simulink model "sampleModel1882"  (R2023a)
settings: Solver=VariableStepAuto  StartTime=0.0  StopTime=10.0  RelTol=1e-3
libraries: hdlsllib x4, simulink x1
settings Model: Creator=user1  LastModifiedBy=user1

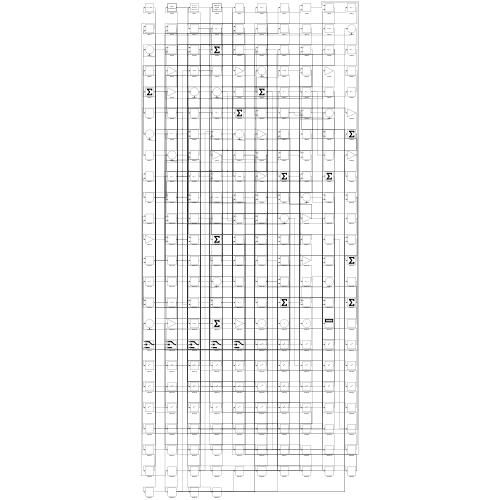
[thumbnail: Simulink's stored preview of the top-level diagram]
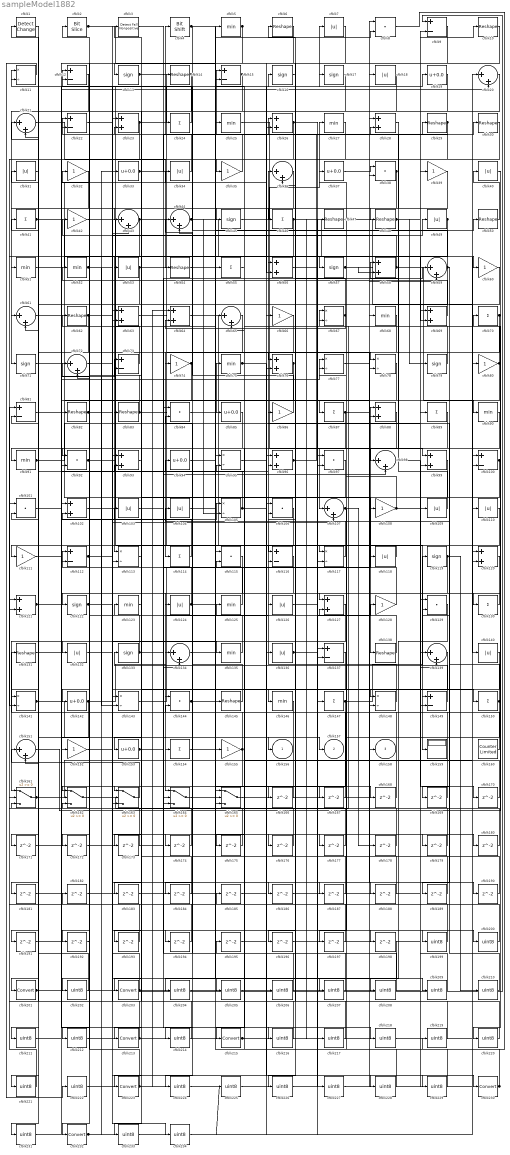
== system sampleModel1882 ==
  cfblk1 : simulink/Logic and Bit Operations/Detect Change  vinit=0  OutDataTypeStr=boolean
      settings: LibrarySourceBlock=|
      | hdlsllib/Logic and Bit
      | Operations/Detect
      | Change
  cfblk{6,10,14,29..30,47..48,50,54,62,82..83,131,138,145} (15 alike) : Reshape
  cfblk{9,12,15,22,73,81,100,112,116,137,149} (11 alike) : Sum  Inputs=+-
  cfblk{8,38,84,92,97,101,106,115,129,144} (10 alike) : DotProduct  OutDataTypeStr=Inherit: Inherit via internal rule
  cfblk{23,26,28,56,58,63..64,69,76,88,93,96,99,102,120..121,127} (17 alike) : Sum
  cfblk{7,18,31,34,40,49,53,103..104,109..110,118,124,126,132,136,140} (17 alike) : Abs  SaturateOnIntegerOverflow=off
  cfblk{11,67,77..78,95,105,113,117,141,143,148} (11 alike) : Product  Inputs=*/  RndMeth=Zero  SaturateOnIntegerOverflow=on
  cfblk{20..21,36,43..44,59,61,65,72,98,107,134,139,151} (14 alike) : Sum  Inputs=|++
  cfblk{32,35,39,42,60,66,74,80,86,108,111,128,152,155} (14 alike) : Gain
  cfblk{24,41,46,55,70,87,89,114,130,147,150,154} (12 alike) : Sum  Inputs=+
  cfblk{13,16..17,45,57,71,79,119,122,133} (10 alike) : Signum
  cfblk{5,25,27,51..52,68,75,90..91,123,125,135,146} (13 alike) : MinMax
  cfblk{19,33,37,85,94,142,153} (7 alike) : Bias  Bias=0.0  SaturateOnIntegerOverflow=off
  cfblk159 : Display
  cfblk160 : hdlsllib/Sources/Counter Limited  uplimit=7  tsamp=-1
  cfblk{161..165} (5 alike) : Switch  SaturateOnIntegerOverflow=off  InputSameDT=off
  cfblk{166..198} (33 alike) : Delay  SampleTime=1
  cfblk{199..200,202,204..212,214,216..222,224..229,231,233..234} (29 alike) : DataTypeConversion  OutDataTypeStr=uint8  SaturateOnIntegerOverflow=off  RndMeth=Floor
  cfblk2 : hdlsllib/Logic and Bit Operations/Bit Slice  lidx=7  ridx=0
  cfblk{201,203,213,215,223,230,232} (7 alike) : DataTypeConversion  SaturateOnIntegerOverflow=off  RndMeth=Floor
  cfblk3 : hdlsllib/Logic and Bit Operations/Detect Fall Nonpositive  vinit=0  OutDataTypeStr=boolean
  cfblk4 : hdlsllib/Logic and Bit Operations/Bit Shift  mode=Shift Left Logical  N=0
  cfblk156 : Outport  VectorParamsAs1DForOutWhenUnconnected=off
  cfblk157 : Outport  Port=2  VectorParamsAs1DForOutWhenUnconnected=off
  cfblk158 : Outport  Port=3  VectorParamsAs1DForOutWhenUnconnected=off
  wires:
  cfblk127/1 -> cfblk161/1
  cfblk58/1 -> cfblk90/1, cfblk42/1
  cfblk42/1 -> cfblk117/1
  cfblk107/1 -> cfblk133/1, cfblk178/1
  cfblk12/1 -> cfblk71/1
  cfblk162/1 -> cfblk67/1
  cfblk96/1 -> cfblk30/1, cfblk196/1
  cfblk10/1 -> cfblk13/1
  cfblk50/1 -> cfblk40/1
  cfblk5/1 -> cfblk122/1, cfblk112/2
  cfblk150/1 -> cfblk86/1, cfblk104/1, cfblk197/1
  cfblk91/1 -> cfblk88/1, cfblk9/2, cfblk96/2
  cfblk25/1 -> cfblk99/1
  cfblk64/1 -> cfblk159/1
  cfblk151/1 -> cfblk70/1
  cfblk49/1 -> cfblk113/1, cfblk69/2
  cfblk71/1 -> cfblk138/1
  cfblk92/1 -> cfblk7/1, cfblk14/1
  cfblk17/1 -> cfblk132/1
  cfblk66/1 -> cfblk114/1
  cfblk148/1 -> cfblk36/1
  cfblk124/1 -> cfblk5/1, cfblk73/2
  cfblk40/1 -> cfblk130/1
  cfblk84/1 -> cfblk75/1
  cfblk80/1 -> cfblk22/1, cfblk148/2
  cfblk145/1 -> cfblk102/2
  cfblk141/1 -> cfblk157/1, cfblk77/2
  cfblk134/1 -> cfblk65/1
  cfblk120/1 -> cfblk232/1
  cfblk163/1 -> cfblk151/1
  cfblk106/1 -> cfblk215/1
  cfblk44/1 -> cfblk57/1, cfblk105/2
  cfblk117/1 -> cfblk56/1
  cfblk114/1 -> cfblk32/1
  cfblk119/1 -> cfblk164/1, cfblk210/1
  cfblk142/1 -> cfblk126/1, cfblk191/1
  cfblk54/1 -> cfblk55/1
  cfblk94/1 -> cfblk155/1
  cfblk147/1 -> cfblk119/1, cfblk192/1
  cfblk7/1 -> cfblk146/1
  cfblk83/1 -> cfblk165/1, cfblk62/1
  cfblk102/1 -> cfblk50/1
  cfblk34/1 -> cfblk4/1
  cfblk47/1 -> cfblk100/1
  cfblk133/1 -> cfblk112/1, cfblk177/1
  cfblk43/1 -> cfblk78/1, cfblk141/2
  cfblk165/1 -> cfblk8/1
  cfblk45/1 -> cfblk27/1
  cfblk23/1 -> cfblk16/1, cfblk121/2
  cfblk13/1 -> cfblk76/1, cfblk216/1
  cfblk152/1 -> cfblk230/1
  cfblk41/1 -> cfblk117/2, cfblk97/2
  cfblk19/1 -> cfblk63/2
  cfblk115/1 -> cfblk203/1
  cfblk121/1 -> cfblk154/1, cfblk34/1, cfblk105/1
  cfblk137/1 -> cfblk223/1
  cfblk139/1 -> cfblk148/1
  cfblk95/1 -> cfblk136/1
  cfblk128/1 -> cfblk2/1
  cfblk109/1 -> cfblk24/1
  cfblk122/1 -> cfblk186/1, cfblk187/1
  cfblk153/1 -> cfblk59/1, cfblk118/1
  cfblk143/1 -> cfblk88/2
  cfblk70/1 -> cfblk116/1, cfblk72/2
  cfblk1/1 -> cfblk201/1
  cfblk85/1 -> cfblk113/2
  cfblk2/1 -> cfblk85/1, cfblk194/1
  cfblk100/1 -> cfblk165/2, cfblk220/1
  cfblk62/1 -> cfblk135/1, cfblk181/1
  cfblk53/1 -> cfblk165/3, cfblk98/2, cfblk171/1
  cfblk112/1 -> cfblk49/1, cfblk172/1, cfblk176/1
  cfblk48/1 -> cfblk98/1, cfblk79/1, cfblk10/1
  cfblk38/1 -> cfblk44/2, cfblk183/1
  cfblk93/1 -> cfblk23/2
  cfblk67/1 -> cfblk26/1, cfblk64/2
  cfblk46/1 -> cfblk100/2, cfblk141/1, cfblk217/1
  cfblk21/1 -> cfblk54/1
  cfblk118/1 -> cfblk111/1
  cfblk22/1 -> cfblk108/1
  cfblk37/1 -> cfblk38/1
  cfblk35/1 -> cfblk15/1
  cfblk36/1 -> cfblk45/1
  cfblk155/1 -> cfblk131/1, cfblk184/1
  cfblk87/1 -> cfblk124/1, cfblk59/2
  cfblk154/1 -> cfblk8/2
  cfblk61/1 -> cfblk158/1
  cfblk63/1 -> cfblk145/1
  cfblk144/1 -> cfblk156/1, cfblk209/1
  cfblk130/1 -> cfblk127/1
  cfblk33/1 -> cfblk60/1, cfblk29/1
  cfblk75/1 -> cfblk87/1, cfblk207/1
  cfblk105/1 -> cfblk41/1, cfblk200/1
  cfblk29/1 -> cfblk61/1, cfblk53/1, cfblk28/2
  cfblk51/1 -> cfblk17/1
  cfblk78/1 -> cfblk164/2
  cfblk76/1 -> cfblk83/1, cfblk92/2
  cfblk28/1 -> cfblk48/1
  cfblk69/1 -> cfblk52/1
  cfblk57/1 -> cfblk140/1, cfblk58/2
  cfblk26/1 -> cfblk78/2, cfblk35/1
  cfblk79/1 -> cfblk58/1
  cfblk73/1 -> cfblk12/1
  cfblk52/1 -> cfblk143/2, cfblk174/1
  cfblk24/1 -> cfblk11/1
  cfblk90/1 -> cfblk107/1
  cfblk14/1 -> cfblk43/1, cfblk142/1
  cfblk140/1 -> cfblk164/3
  cfblk101/1 -> cfblk19/1
  cfblk32/1 -> cfblk51/1
  cfblk4/1 -> cfblk134/1, cfblk150/1
  cfblk131/1 -> cfblk20/2
  cfblk160/1 -> cfblk11/2
  cfblk161/1 -> cfblk80/1, cfblk31/1
  cfblk86/1 -> cfblk44/1
  cfblk9/1 -> cfblk46/1
  cfblk27/1 -> cfblk163/3
  cfblk138/1 -> cfblk125/1
  cfblk59/1 -> cfblk61/2, cfblk12/2, cfblk189/1
  cfblk15/1 -> cfblk21/2, cfblk92/1
  cfblk132/1 -> cfblk43/2
  cfblk123/1 -> cfblk213/1
  cfblk135/1 -> cfblk103/1
  cfblk149/1 -> cfblk6/1
  cfblk97/1 -> cfblk144/1
  cfblk108/1 -> cfblk139/1, cfblk67/2, cfblk77/1
  cfblk31/1 -> cfblk91/1
  cfblk55/1 -> cfblk25/1
  cfblk125/1 -> cfblk72/1
  cfblk65/1 -> cfblk74/1
  cfblk111/1 -> cfblk73/1
  cfblk82/1 -> cfblk149/1, cfblk107/2, cfblk205/1
  cfblk74/1 -> cfblk162/1, cfblk153/1
  cfblk136/1 -> cfblk128/1, cfblk229/1
  cfblk6/1 -> cfblk56/2
  cfblk16/1 -> cfblk166/1
  cfblk166/1 -> cfblk163/1
  cfblk110/1 -> cfblk167/1
  cfblk167/1 -> cfblk101/2
  cfblk164/1 -> cfblk168/1
  cfblk168/1 -> cfblk102/1
  cfblk60/1 -> cfblk169/1
  cfblk169/1 -> cfblk116/2
  cfblk98/1 -> cfblk170/1
  cfblk170/1 -> cfblk15/2
  cfblk171/1 -> cfblk134/2
  cfblk113/1 -> cfblk173/1
  cfblk173/1 -> cfblk22/2
  cfblk174/1 -> cfblk163/2
  cfblk88/1 -> cfblk175/1
  cfblk175/1 -> cfblk151/2
  cfblk176/1 -> cfblk65/2
  cfblk177/1 -> cfblk161/2
  cfblk178/1 -> cfblk127/2
  cfblk56/1 -> cfblk179/1
  cfblk179/1 -> cfblk63/1
  cfblk103/1 -> cfblk180/1
  cfblk180/1 -> cfblk21/1
  cfblk181/1 -> cfblk26/2
  cfblk183/1 -> cfblk76/2
  cfblk184/1 -> cfblk93/2
  cfblk186/1 -> cfblk99/2
  cfblk187/1 -> cfblk144/2
  cfblk72/1 -> cfblk188/1
  cfblk188/1 -> cfblk36/2
  cfblk189/1 -> cfblk97/1
  cfblk77/1 -> cfblk190/1
  cfblk190/1 -> cfblk28/1
  cfblk191/1 -> cfblk162/2
  cfblk192/1 -> cfblk162/3
  cfblk18/1 -> cfblk193/1
  cfblk193/1 -> cfblk23/1
  cfblk194/1 -> cfblk161/3
  cfblk196/1 -> cfblk139/2
  cfblk197/1 -> cfblk121/1
  cfblk104/1 -> cfblk198/1
  cfblk3/1 -> cfblk199/1
  cfblk199/1 -> cfblk94/1
  cfblk200/1 -> cfblk3/1
  cfblk201/1 -> cfblk69/1, cfblk109/1
  cfblk182/1 -> cfblk202/1
  cfblk202/1 -> cfblk1/1
  cfblk203/1 -> cfblk9/1, cfblk93/1
  cfblk198/1 -> cfblk204/1
  cfblk204/1 -> cfblk115/1
  cfblk205/1 -> cfblk115/2
  cfblk185/1 -> cfblk206/1
  cfblk206/1 -> cfblk84/1
  cfblk207/1 -> cfblk185/1
  cfblk129/1 -> cfblk208/1
  cfblk208/1 -> cfblk84/2
  cfblk209/1 -> cfblk129/1
  cfblk210/1 -> cfblk129/2
  cfblk89/1 -> cfblk211/1
  cfblk211/1 -> cfblk82/1
  cfblk116/1 -> cfblk212/1
  cfblk212/1 -> cfblk89/1
  cfblk213/1 -> cfblk149/2, cfblk143/1
  cfblk20/1 -> cfblk214/1
  cfblk214/1 -> cfblk123/1
  cfblk215/1 -> cfblk18/1, cfblk147/1
  cfblk216/1 -> cfblk106/1
  cfblk217/1 -> cfblk106/2
  cfblk81/1 -> cfblk218/1
  cfblk218/1 -> cfblk110/1
  cfblk8/1 -> cfblk219/1
  cfblk219/1 -> cfblk81/1
  cfblk220/1 -> cfblk81/2
  cfblk39/1 -> cfblk221/1
  cfblk221/1 -> cfblk101/1
  cfblk11/1 -> cfblk222/1
  cfblk222/1 -> cfblk39/1
  cfblk223/1 -> cfblk182/1, cfblk38/2, cfblk64/1
  cfblk146/1 -> cfblk224/1
  cfblk224/1 -> cfblk137/1
  cfblk225/1 -> cfblk137/2
  cfblk68/1 -> cfblk226/1
  cfblk226/1 -> cfblk20/1
  cfblk126/1 -> cfblk227/1
  cfblk227/1 -> cfblk68/1
  cfblk195/1 -> cfblk228/1
  cfblk228/1 -> cfblk95/1
  cfblk229/1 -> cfblk195/1
  cfblk230/1 -> cfblk95/2, cfblk37/1
  cfblk30/1 -> cfblk231/1
  cfblk231/1 -> cfblk152/1
  cfblk232/1 -> cfblk225/1, cfblk47/1, cfblk96/1, cfblk66/1, cfblk33/1
  cfblk99/1 -> cfblk233/1
  cfblk233/1 -> cfblk120/1
  cfblk172/1 -> cfblk234/1
  cfblk234/1 -> cfblk120/2
